simulink model "sobel_fpga"  (R2013a)
settings: Solver=ode45  StartTime=0.0  StopTime=10000  RelTol=1e-3
undefined symbols (not defined in the file or in its folder): A, gray, N, xlipgetpartsetting
libraries: xbsIndex_r4 x19, dspmtrx3 x6, dspsigattribs x3, visionsinks x3, visionsources x1, xrbsImage_r4 x1, JTAGRuntimeCosim_r4 x1
settings Model: Creator=diegohr  LastModifiedBy=diego

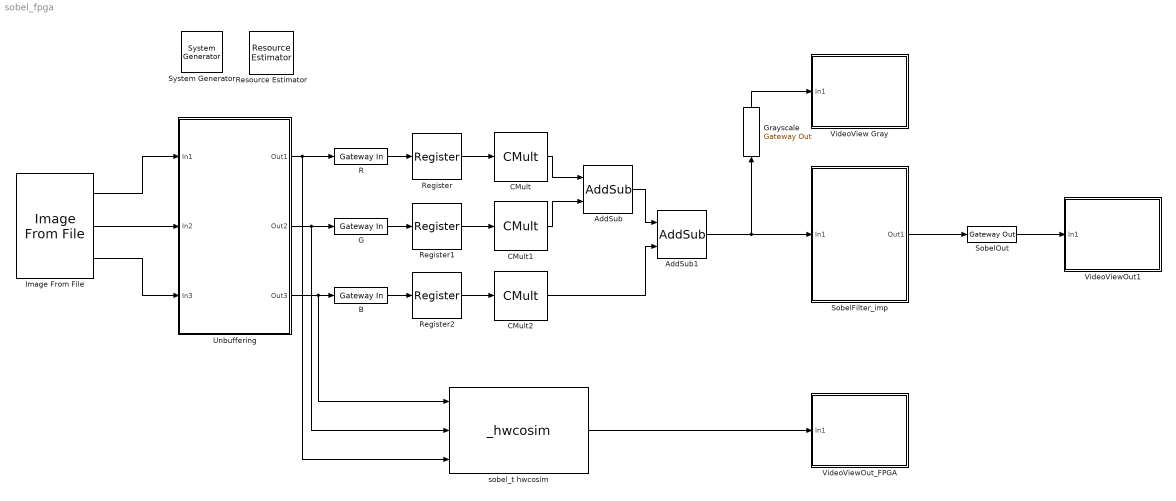
== system sobel_fpga ==
  " System Generator" : xbsIndex_r4/ System Generator  Tag=genX  xilinxfamily=spartan6  part=xc6slx45t  speed=-3  package=fgg484  synthesis_tool=XST  clock_wrapper=Clock Enables  directory=./netlist  proj_type=Project Navigator  Synth_file=XST Defaults  Impl_file=ISE Defaults  testbench=off  simulink_period=5.0863e-06  sysclk_period=15  dcm_input_clock_period=10  incr_netlist=off  trim_vbits=Everywhere in SubSystem  dbl_ovrd=According to Block Masks  core_generation=According to Block Masks  run_coregen=off  deprecated_control=off  eval_field=0  block_type=sysgen
  AddSub : xbsIndex_r4/AddSub  mode=Addition  use_carryin=off  use_carryout=off  en=off  latency=0  precision=Full  arith_type=Unsigned  n_bits=16  bin_pt=14  quantization=Truncate  overflow=Wrap  dbl_ovrd=off  use_behavioral_HDL=off  hw_selection=Fabric  pipelined=off  block_type=addsub
  AddSub1 : xbsIndex_r4/AddSub  mode=Addition  use_carryin=off  use_carryout=off  en=off  latency=0  precision=Full  arith_type=Unsigned  n_bits=16  bin_pt=14  quantization=Truncate  overflow=Wrap  dbl_ovrd=off  use_behavioral_HDL=off  hw_selection=Fabric  pipelined=off  block_type=addsub
  B : xbsIndex_r4/Gateway In  gui_display_data_type=Fixed-point  arith_type=Unsigned  n_bits=16  bin_pt=14  preci_type=Single  exp_width=8  frac_width=24  quantization="Round  (unbiased: +/- Inf)"  overflow=Saturate  period=5.0863e-06  dbl_ovrd=off  timing_constraint=None  locs_specified=off  LOCs={}  UseAsADC=off  ADCChannel='1'  inherit_from_input=off  hdl_port=on  block_type=gatewayin
  CMult : xbsIndex_r4/CMult  const=0.2989  gui_display_data_type=Fixed-point  const_n_bits=16  const_bin_pt=14  float_type=Single  exp_bits=8  fraction_bits=24  en=off  latency=0  precision=Full  arith_type="Signed  (2's comp)"  n_bits=16  bin_pt=14  quantization=Truncate  overflow=Wrap  dbl_ovrd=off  use_behavioral_HDL=off  mem_type=Distributed RAM  pipeline=off  block_type=cmult
  CMult1 : xbsIndex_r4/CMult  const=0.5870  gui_display_data_type=Fixed-point  const_n_bits=16  const_bin_pt=14  float_type=Single  exp_bits=8  fraction_bits=24  en=off  latency=0  precision=Full  arith_type="Signed  (2's comp)"  n_bits=16  bin_pt=14  quantization=Truncate  overflow=Wrap  dbl_ovrd=off  use_behavioral_HDL=off  mem_type=Distributed RAM  pipeline=off  block_type=cmult
  CMult2 : xbsIndex_r4/CMult  const=0.1140  gui_display_data_type=Fixed-point  const_n_bits=16  const_bin_pt=14  float_type=Single  exp_bits=8  fraction_bits=24  en=off  latency=0  precision=Full  arith_type="Signed  (2's comp)"  n_bits=16  bin_pt=14  quantization=Truncate  overflow=Wrap  dbl_ovrd=off  use_behavioral_HDL=off  mem_type=Distributed RAM  pipeline=off  block_type=cmult
  G : xbsIndex_r4/Gateway In  gui_display_data_type=Fixed-point  arith_type=Unsigned  n_bits=16  bin_pt=14  preci_type=Single  exp_width=8  frac_width=24  quantization="Round  (unbiased: +/- Inf)"  overflow=Saturate  period=5.0863e-06  dbl_ovrd=off  timing_constraint=None  locs_specified=off  LOCs={}  UseAsADC=off  ADCChannel='1'  inherit_from_input=off  hdl_port=on  block_type=gatewayin
  Grayscale : xbsIndex_r4/Gateway Out  inherit_from_input=off  hdl_port=off  timing_constraint=None  locs_specified=off  LOCs={}  UseAsDAC=off  DACChannel='1'  block_type=gatewayout
  Image From File : visionsources/Image From File  Tag=vipblks_nd  FileName=peppers.png  imagePorts=Separate color signals  Ts=inf  ImageDataType=double  Signed=on  WordLength=16  sdImageDataType=uint(8)  FractionLengthMode=User-defined  FractionLength=15  OutPortLabels=R|G|B
  R : xbsIndex_r4/Gateway In  gui_display_data_type=Fixed-point  arith_type=Unsigned  n_bits=16  bin_pt=14  preci_type=Single  exp_width=8  frac_width=24  quantization="Round  (unbiased: +/- Inf)"  overflow=Saturate  period=5.0863e-06  dbl_ovrd=off  timing_constraint=None  locs_specified=off  LOCs={}  UseAsADC=off  ADCChannel='1'  inherit_from_input=off  hdl_port=on  block_type=gatewayin
  Register : xbsIndex_r4/Register  init=0  rst=off  en=off  dbl_ovrd=off  block_type=register
  Register1 : xbsIndex_r4/Register  init=0  rst=off  en=off  dbl_ovrd=off  block_type=register
  Register2 : xbsIndex_r4/Register  init=0  rst=off  en=off  dbl_ovrd=off  block_type=register
  Resource Estimator : xbsIndex_r4/Resource Estimator  Tag=resEstTag  Slices=0  FFs=0  BRAMs=0  LUTs=0  IOBs=0  EBMs=0  TBUFs=0  xl_use_estimator_area=off  est_options=Post Map  block_type=resource_estimator
      settings: AttributesFormatString=Resource\nEstimator
  SobelFilter_imp : Subsystem
  SobelOut : xbsIndex_r4/Gateway Out  inherit_from_input=off  hdl_port=on  timing_constraint=None  locs_specified=off  LOCs={}  UseAsDAC=off  DACChannel='1'  block_type=gatewayout
  Unbuffering : Subsystem
  VideoView Gray : Subsystem
  VideoViewOut1 : Subsystem
  VideoViewOut_FPGA : Subsystem
  sobel_t hwcosim : JTAGRuntimeCosim_r4/_hwcosim  clkSrc=Single Stepped  hasCombinationalPath=on  bitfileName=/home/diego/Documents/Finalized/examples/sobel_img/netlist/sobel_t_cw.bit  skipConfig=off  cable=Auto Detect  speed=N/A  cablePort=N/A  cableLocation=Local  shareCable=on  enable_codebug=on  design_xtable=|  engineDll=JTAGCosimEngine.dll  cableWaitTime=10  bscanPos=-1  IRLengths=[]  useWaitBox=1  hasBufgmux=on  Scheme=Cosim  useCmdProc=1  hasProc=0  useImpact=0  printLogFile=0  block_type=jtagcosim
      | {
      |   'clkWrapper' => 'sobel_t_cw',
      |   'clocksGcd' => 1,
      |   'device' => 'xc6slx45t-3fgg484',
      |   'ports' => {
      |     'b' => {
      |       'bd_port_index' => 0,
      |       'direction' => 'in',
      |       'icon_text' => 'B',
      |       'period' => 1,
      |       'sim_pause_trigger' => false,
      |       'type' => 'UFix_16_14',
      |       'width' => 16,
      |     },
      |     'g' => {
      |       'bd_port_index' => 1,
      |       'direction' => 'in',
      |       'icon_text' => 'G',
      |       'period' => 1,
      |       'sim_pause_trigger' => false,
      |       'type' => 'UFix_16_14',
      |       'width' => 16,
      |     },
      |     'r' => {
      |       'bd_port_index' => 2,
      |       'direction' => 'in',
      |       'icon_text' => 'R',
      |       'period' => 1,
      |       'sim_pause_trigger' => false,
      |       'type' => 'UFix_16_14',
      |       'width' => 16,
      |     },
      |     'sobelout' => {
      |       'bd_port_index' => 0,
      |       'direction' => 'out',
      |       'icon_text' => 'SobelOut',
      |       'period' => 1,
      |       'sim_pause_trigger' => false,
      |       'type' => 'Fix_41_28',
      |       'width' => 41,
      |     },
      |   },
      |   'shared_memories' => {},
      | }
  wires:
  Image From File/2 -> Unbuffering/2(In2)
  Image From File/1 -> Unbuffering/1(In1)
  Image From File/3 -> Unbuffering/3(In3)
  Unbuffering/2(Out2) -> sobel_t hwcosim/2, G/1
  Unbuffering/1(Out1) -> sobel_t hwcosim/3, R/1
  Unbuffering/3(Out3) -> sobel_t hwcosim/1, B/1
  R/1 -> Register/1
  G/1 -> Register1/1
  B/1 -> Register2/1
  Register/1 -> CMult/1
  Register1/1 -> CMult1/1
  Register2/1 -> CMult2/1
  CMult/1 -> AddSub/1
  CMult1/1 -> AddSub/2
  CMult2/1 -> AddSub1/2
  AddSub/1 -> AddSub1/1
  Grayscale/1 -> VideoView Gray/1(In1)
  SobelOut/1 -> VideoViewOut1/1(In1)
  SobelFilter_imp/1(Out1) -> SobelOut/1
  AddSub1/1 -> Grayscale/1, SobelFilter_imp/1(In1)
  sobel_t hwcosim/1 -> VideoViewOut_FPGA/1(In1)

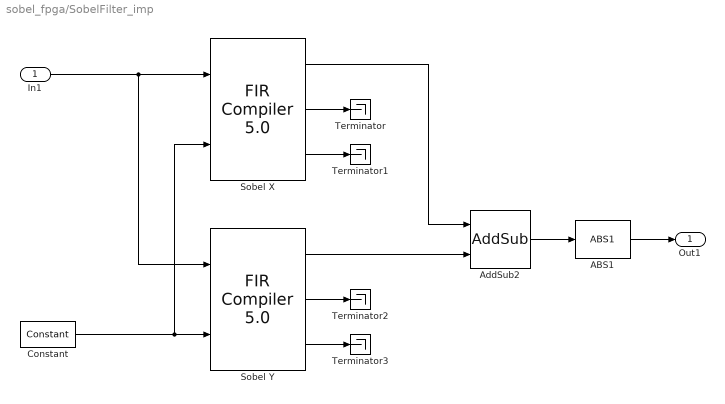
== system sobel_fpga/SobelFilter_imp ==
  In1 : Inport
  ABS1 : xrbsImage_r4/5x5Filter/ABS1
  AddSub2 : xbsIndex_r4/AddSub  mode=Addition  use_carryin=off  use_carryout=off  en=off  latency=0  precision=Full  arith_type=Unsigned  n_bits=16  bin_pt=14  quantization=Truncate  overflow=Wrap  dbl_ovrd=off  use_behavioral_HDL=off  hw_selection=Fabric  pipelined=off  block_type=addsub
  Constant : xbsIndex_r4/Constant  const=1  gui_display_data_type=Boolean  arith_type=Boolean  n_bits=16  bin_pt=14  preci_type=Single  exp_width=8  frac_width=24  explicit_period=off  period=1  equ=P=C  opselect=C  inp2=PCIN>>17  opr=+  inp1=P  carry=CIN  dbl_ovrd=off  block_type=constant
  Sobel X : xbsIndex_r4/FIR Compiler 5.0   coefficientvector=[-1, 0, +1, -2, 0, +2, -1, 0, +1]  coefficient_sets=1  filter_type=Single_Rate  rate_change_type=Integer  interpolation_rate=1  decimation_rate=1  zero_pack_factor=1  number_channels=1  ratespecification=Sample_Period  sampleperiod=1  hardwareoversamplingrate=1  filter_architecture=Transpose_Multiply_Accumulate  coefficient_reload=off  coefficient_structure=Inferred  coefficient_sign=Signed  quantization=Integer_Coefficients  coefficient_width=16  bestprecision=off  coefficient_fractional_bits=0  number_paths=1  output_rounding_mode=Full_Precision  output_width=20  allow_rounding_approximation=off  optimization_goal=Area  has_sclr=off  has_data_valid=off  has_nd=on  has_ce=off  usechan_in_adv=off  chan_in_adv=0  data_buffer_type=Not_Applicable  coefficient_buffer_type=Not_Applicable  input_buffer_type=Not_Applicable  output_buffer_type=Not_Applicable  preference_for_other_storage=Not_Applicable  multi_column_support=Disabled  columnconfig='9'  inter_column_pipe_length=4  passband_min=0.0  passband_max=0.5  stopband_min=0.5  stopband_max=1.0  filter_selection=1  gui_behaviour=Sysgen  registered_output=true  data_sign=Signed  data_width=16  data_fractional_bits=0  wrapper_available=true  ip_wrap_arbitrary_binary_point=true  ip_name=FIR Compiler  ip_version=5.0  dsptool_ready=true  ipcore_usecache=true  ipcore_useipmodelcache=true  ipcore_xco_need_fpga_part=true  port_translation_map={ 'ce' => 'en', 'sclr' => 'rst' }  run_core_at_system_period=true  ipcore_fpga_part=xlipgetpartsetting(gcb, {'virtex4', 'xc4vsx35', '-10', 'ff668'})  structural_sim=false  block_type=fir_compiler_v5_0
  Sobel Y : xbsIndex_r4/FIR Compiler 5.0   coefficientvector=[+1, +2, +1, 0, 0, 0, -1, -2, -1]  coefficient_sets=1  filter_type=Single_Rate  rate_change_type=Integer  interpolation_rate=1  decimation_rate=1  zero_pack_factor=1  number_channels=1  ratespecification=Sample_Period  sampleperiod=1  hardwareoversamplingrate=1  filter_architecture=Transpose_Multiply_Accumulate  coefficient_reload=off  coefficient_structure=Inferred  coefficient_sign=Signed  quantization=Integer_Coefficients  coefficient_width=16  bestprecision=off  coefficient_fractional_bits=0  number_paths=1  output_rounding_mode=Full_Precision  output_width=20  allow_rounding_approximation=off  optimization_goal=Area  has_sclr=off  has_data_valid=off  has_nd=on  has_ce=off  usechan_in_adv=off  chan_in_adv=0  data_buffer_type=Not_Applicable  coefficient_buffer_type=Not_Applicable  input_buffer_type=Not_Applicable  output_buffer_type=Not_Applicable  preference_for_other_storage=Not_Applicable  multi_column_support=Disabled  columnconfig='9'  inter_column_pipe_length=4  passband_min=0.0  passband_max=0.5  stopband_min=0.5  stopband_max=1.0  filter_selection=1  gui_behaviour=Sysgen  registered_output=true  data_sign=Signed  data_width=16  data_fractional_bits=0  wrapper_available=true  ip_wrap_arbitrary_binary_point=true  ip_name=FIR Compiler  ip_version=5.0  dsptool_ready=true  ipcore_usecache=true  ipcore_useipmodelcache=true  ipcore_xco_need_fpga_part=true  port_translation_map={ 'ce' => 'en', 'sclr' => 'rst' }  run_core_at_system_period=true  ipcore_fpga_part=xlipgetpartsetting(gcb, {'virtex4', 'xc4vsx35', '-10', 'ff668'})  structural_sim=false  block_type=fir_compiler_v5_0
  Terminator{,1..3} (4 alike) : Terminator
  Out1 : Outport
  wires:
  Constant/1 -> Sobel X/2, Sobel Y/2
  In1/1 -> Sobel Y/1, Sobel X/1
  Sobel X/2 -> Terminator/1
  Sobel X/3 -> Terminator1/1
  Sobel Y/2 -> Terminator2/1
  Sobel Y/3 -> Terminator3/1
  Sobel X/1 -> AddSub2/1
  Sobel Y/1 -> AddSub2/2
  AddSub2/1 -> ABS1/1
  ABS1/1 -> Out1/1

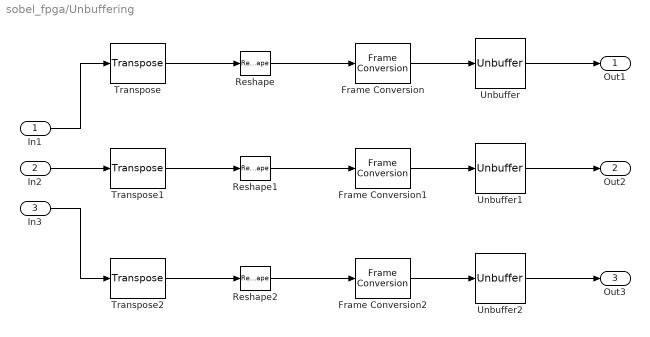
== system sobel_fpga/Unbuffering ==
  In1 : Inport
  In2 : Inport  Port=2
  In3 : Inport  Port=3
  Frame Conversion : FrameConversion
  Frame Conversion1 : FrameConversion
  Frame Conversion2 : FrameConversion
  Reshape : Reshape
  Reshape1 : Reshape
  Reshape2 : Reshape
  Transpose : dspmtrx3/Transpose  Hermitian=off  overflowFlag=off
  Transpose1 : dspmtrx3/Transpose  Hermitian=off  overflowFlag=off
  Transpose2 : dspmtrx3/Transpose  Hermitian=off  overflowFlag=off
  Unbuffer : Unbuffer  SampleBasedProcessing=Same as frame based
  Unbuffer1 : Unbuffer  SampleBasedProcessing=Same as frame based
  Unbuffer2 : Unbuffer  SampleBasedProcessing=Same as frame based
  Out1 : Outport
  Out2 : Outport  Port=2
  Out3 : Outport  Port=3
  wires:
  In1/1 -> Transpose/1
  In3/1 -> Transpose2/1
  Reshape2/1 -> Frame Conversion2/1
  Frame Conversion1/1 -> Unbuffer1/1
  Transpose/1 -> Reshape/1
  Unbuffer/1 -> Out1/1
  Reshape1/1 -> Frame Conversion1/1
  Transpose2/1 -> Reshape2/1
  Reshape/1 -> Frame Conversion/1
  Unbuffer1/1 -> Out2/1
  Unbuffer2/1 -> Out3/1
  Frame Conversion/1 -> Unbuffer/1
  Frame Conversion2/1 -> Unbuffer2/1
  In2/1 -> Transpose1/1
  Transpose1/1 -> Reshape1/1

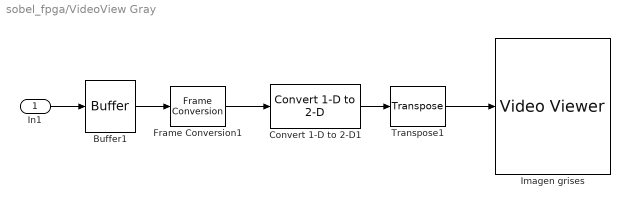
== system sobel_fpga/VideoView Gray ==
  In1 : Inport
  Buffer1 : Buffer  N=196608  TreatMby1Signals=One channel
  Convert 1-D to 2-D1 : dspsigattribs/Convert 1-D to 2-D  M=512  N=384  frameBasedOut=off
  Frame Conversion1 : FrameConversion
  Imagen grises : visionsinks/Video Viewer  inputType=Obsolete7b  imagePorts=One multidimensional signal  useColorMap=off  colormapValue=gray(256)  specRange=off  minInputVal=0  maxInputVal=255  FigPos=[439 705 742 513]  AxisZoom=on  trueSizedOnce=off  OpenAtMdlStart=on  DefaultConfigurationName=vipscopes.VideoViewerScopeCfg
  Transpose1 : dspmtrx3/Transpose  Hermitian=off  overflowFlag=off
  wires:
  Convert 1-D to 2-D1/1 -> Transpose1/1
  Buffer1/1 -> Frame Conversion1/1
  Frame Conversion1/1 -> Convert 1-D to 2-D1/1
  Transpose1/1 -> Imagen grises/1
  In1/1 -> Buffer1/1

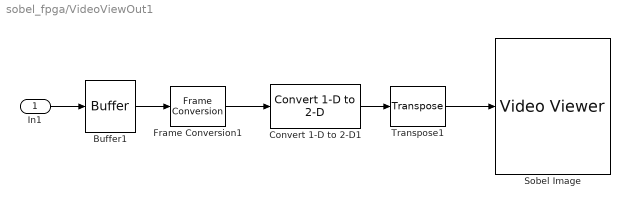
== system sobel_fpga/VideoViewOut1 ==
  In1 : Inport
  Buffer1 : Buffer  N=196608  TreatMby1Signals=One channel
  Convert 1-D to 2-D1 : dspsigattribs/Convert 1-D to 2-D  M=512  N=384  frameBasedOut=off
  Frame Conversion1 : FrameConversion
  Sobel Image : visionsinks/Video Viewer  inputType=Obsolete7b  imagePorts=One multidimensional signal  useColorMap=off  colormapValue=gray(256)  specRange=off  minInputVal=0  maxInputVal=255  FigPos=[582 677 742 513]  AxisZoom=on  trueSizedOnce=off  OpenAtMdlStart=on  DefaultConfigurationName=vipscopes.VideoViewerScopeCfg
  Transpose1 : dspmtrx3/Transpose  Hermitian=off  overflowFlag=off
  wires:
  Convert 1-D to 2-D1/1 -> Transpose1/1
  Buffer1/1 -> Frame Conversion1/1
  Frame Conversion1/1 -> Convert 1-D to 2-D1/1
  Transpose1/1 -> Sobel Image/1
  In1/1 -> Buffer1/1

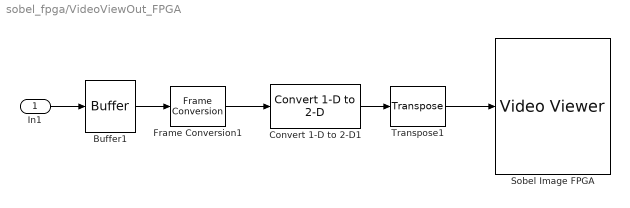
== system sobel_fpga/VideoViewOut_FPGA ==
  In1 : Inport
  Buffer1 : Buffer  N=196608  TreatMby1Signals=One channel
  Convert 1-D to 2-D1 : dspsigattribs/Convert 1-D to 2-D  M=512  N=384  frameBasedOut=off
  Frame Conversion1 : FrameConversion
  Sobel Image FPGA : visionsinks/Video Viewer  inputType=Obsolete7b  imagePorts=One multidimensional signal  useColorMap=off  colormapValue=gray(256)  specRange=off  minInputVal=0  maxInputVal=255  FigPos=[1 662 742 513]  AxisZoom=on  trueSizedOnce=off  OpenAtMdlStart=on  DefaultConfigurationName=vipscopes.VideoViewerScopeCfg
  Transpose1 : dspmtrx3/Transpose  Hermitian=off  overflowFlag=off
  wires:
  Convert 1-D to 2-D1/1 -> Transpose1/1
  Buffer1/1 -> Frame Conversion1/1
  Frame Conversion1/1 -> Convert 1-D to 2-D1/1
  Transpose1/1 -> Sobel Image FPGA/1
  In1/1 -> Buffer1/1
